simulink model "buck_nncontroller_4_10"  (R2021a)
settings: Solver=VariableStepAuto  StartTime=0.0  StopTime=10.0  RelTol=1e-3
libraries: neural x46
(part 2 of 2)

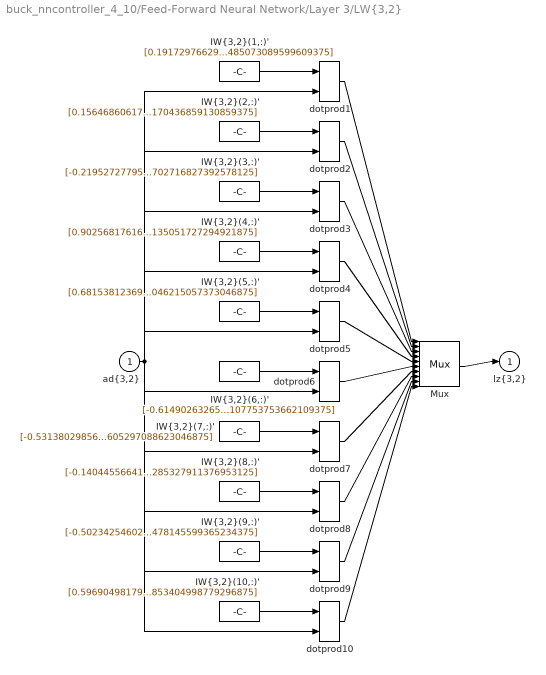
== system buck_nncontroller_4_10/Feed-Forward Neural Network/Layer 3/LW{3,2} ==
  "ad{3,2}" : Inport  PortDimensions=10
      mask Display: e = 0.06;c1 = [120 230 180]/255;c2 = ([120 230 180]+0)/(256+128);c3 = ([120 230 180]+128)/(256+128);patch([0 1 1 0],[0 0 1 1],c1);patch([0 1 1 1-e 1-e 0+e],[0 0 1 1-e 0+e 0+e],c2);patch([0 0 1 1-e 0+e 0+e],[0 1 1 1-e 1-e 0+e],c3);plot([0 1 1 0 0],[0 0 1 1 0]);
  "IW{3,2}(1,:)'" : Constant  Value=[0.19172976629265736647766971145756542682647705078125;0.88614051489335354805376709919073618948459625244140625;0.29738999696942480799322083839797414839267730712890625;-0.25951661377123258489518775604665279388427734375;0.636841676728274297403231685166247189044952392578125;0.11710841092250699746468711737179546616971492767333984375;0.2597575127114775117576073171221651136875152587890625;0.060654299689273917517429168810849660076200962066650390625;-0.0913009511616575952785979097825475037097930908203125;-0.5506828097373277497439403305179439485073089599609375]
      mask Display: e = 0.06;c1 = [120 150 230]/255;c2 = ([120 150 230]+0)/383;c3 = ([120 150 230]+128)/383;patch([0 1 1 0],[0 0 1 1],c1);patch([0 1 1 1-e 1-e 0+e],[0 0 1 1-e 0+e 0+e],c2);patch([0 0 1 1-e 0+e 0+e],[0 1 1 1-e 1-e 0+e],c3);plot([0 1 1 0 0],[0 0 1 1 0]);disp('weights');
  "IW{3,2}(10,:)'" : Constant  Value=[0.5969049817915690336889156242250464856624603271484375;0.76577332732707914519920677776099182665348052978515625;0.96800335487914923593422145131626166403293609619140625;1.0105795441501628229019615901052020490169525146484375;-0.58517005023753465575708787582698278129100799560546875;-0.8478481415545384702880937766167335212230682373046875;0.451249633924208470858729924657382071018218994140625;-0.2305886896661824836396448290543048642575740814208984375;-1.013405147725457755569777873461134731769561767578125;0.1837926427842561938330590010082232765853404998779296875]
      mask Display: e = 0.06;c1 = [120 150 230]/255;c2 = ([120 150 230]+0)/383;c3 = ([120 150 230]+128)/383;patch([0 1 1 0],[0 0 1 1],c1);patch([0 1 1 1-e 1-e 0+e],[0 0 1 1-e 0+e 0+e],c2);patch([0 0 1 1-e 0+e 0+e],[0 1 1 1-e 1-e 0+e],c3);plot([0 1 1 0 0],[0 0 1 1 0]);disp('weights');
  "IW{3,2}(2,:)'" : Constant  Value=[0.1564686061716848985980732322786934673786163330078125;0.06896616915488341936768534878865466453135013580322265625;-0.0680372864971623136920442220798577181994915008544921875;0.243104097467363888807057037411141209304332733154296875;0.53293353025407508294364333778503350913524627685546875;0.39713407865833205701022734501748345792293548583984375;-0.3288549195202807862159488649922423064708709716796875;0.69938333557629539516398153864429332315921783447265625;0.09546105548873760893169304608818492852151393890380859375;0.5713230777177569219560382407507859170436859130859375]
      mask Display: e = 0.06;c1 = [120 150 230]/255;c2 = ([120 150 230]+0)/383;c3 = ([120 150 230]+128)/383;patch([0 1 1 0],[0 0 1 1],c1);patch([0 1 1 1-e 1-e 0+e],[0 0 1 1-e 0+e 0+e],c2);patch([0 0 1 1-e 0+e 0+e],[0 1 1 1-e 1-e 0+e],c3);plot([0 1 1 0 0],[0 0 1 1 0]);disp('weights');
  "IW{3,2}(3,:)'" : Constant  Value=[-0.219527277954874922016870186780579388141632080078125;0.230423420473848505896086180655402131378650665283203125;0.2905036955773778739597901221713982522487640380859375;0.81717580001167167136344460232066921889781951904296875;-0.87206226032498757039235215415828861296176910400390625;-0.35747745545573750280965441561420448124408721923828125;-0.1538746761791760508941706575569696724414825439453125;-0.789495473726509633394243792281486093997955322265625;-0.8454780951510991737762878983630798757076263427734375;-0.5358109195742191133149390225298702716827392578125]
      mask Display: e = 0.06;c1 = [120 150 230]/255;c2 = ([120 150 230]+0)/383;c3 = ([120 150 230]+128)/383;patch([0 1 1 0],[0 0 1 1],c1);patch([0 1 1 1-e 1-e 0+e],[0 0 1 1-e 0+e 0+e],c2);patch([0 0 1 1-e 0+e 0+e],[0 1 1 1-e 1-e 0+e],c3);plot([0 1 1 0 0],[0 0 1 1 0]);disp('weights');
  "IW{3,2}(4,:)'" : Constant  Value=[0.902568176167927394004664165549911558628082275390625;-0.966608055972634883090677249128930270671844482421875;0.630253755399056370123389569926075637340545654296875;-0.07144541546023486233707444625906646251678466796875;0.4724929203673287059217500427621416747570037841796875;-0.564686564149328606987410239526070654392242431640625;-0.393401102039569128265839026425965130329132080078125;0.2267748796151274337518088941578753292560577392578125;-0.116722115632291068010317758307792246341705322265625;0.136222631124105486577491319621913135051727294921875]
      mask Display: e = 0.06;c1 = [120 150 230]/255;c2 = ([120 150 230]+0)/383;c3 = ([120 150 230]+128)/383;patch([0 1 1 0],[0 0 1 1],c1);patch([0 1 1 1-e 1-e 0+e],[0 0 1 1-e 0+e 0+e],c2);patch([0 0 1 1-e 0+e 0+e],[0 1 1 1-e 1-e 0+e],c3);plot([0 1 1 0 0],[0 0 1 1 0]);disp('weights');
  "IW{3,2}(5,:)'" : Constant  Value=[0.6815381236933812925116171754780225455760955810546875;0.8746565583833587620432581388740800321102142333984375;0.92166940991114609804668589276843704283237457275390625;-0.2476291743165152936523298876636545173823833465576171875;0.037965933048799298255016054781663115136325359344482421875;-0.250385559363905552121565278866910375654697418212890625;-0.885720177461852387068574898876249790191650390625;0.71503080156637544018138896717573516070842742919921875;-0.644137823209688153980323477298952639102935791015625;-0.6259347426644552569996449165046215057373046875]
      mask Display: e = 0.06;c1 = [120 150 230]/255;c2 = ([120 150 230]+0)/383;c3 = ([120 150 230]+128)/383;patch([0 1 1 0],[0 0 1 1],c1);patch([0 1 1 1-e 1-e 0+e],[0 0 1 1-e 0+e 0+e],c2);patch([0 0 1 1-e 0+e 0+e],[0 1 1 1-e 1-e 0+e],c3);plot([0 1 1 0 0],[0 0 1 1 0]);disp('weights');
  "IW{3,2}(6,:)'" : Constant  Value=[-0.61490263265205502563048867159523069858551025390625;0.92110822922200774609535756098921410739421844482421875;-0.44997050761879109348484462316264398396015167236328125;0.282435962239532212247894449319574050605297088623046875;0.010975214214938917856034805708986823447048664093017578125;0.24119304606606106755606333535979501903057098388671875;-0.49113879152329165123092025169171392917633056640625;-0.005041658296727861109098878245049490942619740962982177734375;0.7344648388905927749448210306582041084766387939453125;0.606833883210716518163962973630987107753753662109375]
      mask Display: e = 0.06;c1 = [120 150 230]/255;c2 = ([120 150 230]+0)/383;c3 = ([120 150 230]+128)/383;patch([0 1 1 0],[0 0 1 1],c1);patch([0 1 1 1-e 1-e 0+e],[0 0 1 1-e 0+e 0+e],c2);patch([0 0 1 1-e 0+e 0+e],[0 1 1 1-e 1-e 0+e],c3);plot([0 1 1 0 0],[0 0 1 1 0]);disp('weights');
  "IW{3,2}(7,:)'" : Constant  Value=[-0.5313802985629105801734795022639445960521697998046875;-0.2285947124685394349352662857199902646243572235107421875;0.81251823142078982709080037238891236484050750732421875;-0.494273674969173237858655056697898544371128082275390625;-0.28274853484236628364811849678517319262027740478515625;0.80469158884274250009838169717113487422466278076171875;0.2726953250293238095736114701139740645885467529296875;0.314188716095926690030637473682872951030731201171875;-0.351605817074781390463300567716942168772220611572265625;0.3301394158455064342660989495925605297088623046875]
      mask Display: e = 0.06;c1 = [120 150 230]/255;c2 = ([120 150 230]+0)/383;c3 = ([120 150 230]+128)/383;patch([0 1 1 0],[0 0 1 1],c1);patch([0 1 1 1-e 1-e 0+e],[0 0 1 1-e 0+e 0+e],c2);patch([0 0 1 1-e 0+e 0+e],[0 1 1 1-e 1-e 0+e],c3);plot([0 1 1 0 0],[0 0 1 1 0]);disp('weights');
  "IW{3,2}(8,:)'" : Constant  Value=[-0.14044556641976502220359179773367941379547119140625;-0.8208868364874579715007030245033092796802520751953125;-0.9958314486691788314232098855427466332912445068359375;-0.791438289186685128839826575131155550479888916015625;0.984569454586398773443534082616679370403289794921875;-0.498594582463642410630200174637138843536376953125;-0.220996040017324535398302032263018190860748291015625;-0.2023723284278702294614049606025218963623046875;-0.3323634693728434452708597746095620095729827880859375;0.98926969805567654958622370031662285327911376953125]
      mask Display: e = 0.06;c1 = [120 150 230]/255;c2 = ([120 150 230]+0)/383;c3 = ([120 150 230]+128)/383;patch([0 1 1 0],[0 0 1 1],c1);patch([0 1 1 1-e 1-e 0+e],[0 0 1 1-e 0+e 0+e],c2);patch([0 0 1 1-e 0+e 0+e],[0 1 1 1-e 1-e 0+e],c3);plot([0 1 1 0 0],[0 0 1 1 0]);disp('weights');
  "IW{3,2}(9,:)'" : Constant  Value=[-0.50234254602555328261814793222583830356597900390625;-0.67289152066819546416098773988778702914714813232421875;0.80197319581479942218749101812136359512805938720703125;-0.84883813074611536020341873154393397271633148193359375;0.3860056246360417109286800041445530951023101806640625;-0.41908314676562341549725942968507297337055206298828125;-0.00353167369045337409261264838278293609619140625;0.453243465761014707737786011421121656894683837890625;-0.016959986721964082079239233280532062053680419921875;-0.0883321136996553235576357110403478145599365234375]
      mask Display: e = 0.06;c1 = [120 150 230]/255;c2 = ([120 150 230]+0)/383;c3 = ([120 150 230]+128)/383;patch([0 1 1 0],[0 0 1 1],c1);patch([0 1 1 1-e 1-e 0+e],[0 0 1 1-e 0+e 0+e],c2);patch([0 0 1 1-e 0+e 0+e],[0 1 1 1-e 1-e 0+e],c3);plot([0 1 1 0 0],[0 0 1 1 0]);disp('weights');
  Mux : Mux  Inputs=10
      mask Display: e = 0.06;c1 = [120 150 230]/255;c2 = ([120 150 230]+0)/383;c3 = ([120 150 230]+128)/383;patch([0 1 1 0],[0 0 1 1],c1);patch([0 1 1 1-e 1-e 0+e],[0 0 1 1-e 0+e 0+e],c2);patch([0 0 1 1-e 0+e 0+e],[0 1 1 1-e 1-e 0+e],c3);plot([0 1 1 0 0],[0 0 1 1 0]);disp('Mux');
  dotprod{1..10} (10 alike) : neural/Weight Functions/dotprod
  "lz{3,2}" : Outport
      mask Display: e = 0.06;c1 = [120 230 180]/255;c2 = ([120 230 180]+0)/(256+128);c3 = ([120 230 180]+128)/(256+128);patch([0 1 1 0],[0 0 1 1],c1);patch([0 1 1 1-e 1-e 0+e],[0 0 1 1-e 0+e 0+e],c2);patch([0 0 1 1-e 0+e 0+e],[0 1 1 1-e 1-e 0+e],c3);plot([0 1 1 0 0],[0 0 1 1 0]);
  wires:
  "IW{3,2}(1,:)'"/1 -> dotprod1/1
  "ad{3,2}"/1 -> dotprod1/2, dotprod2/2, dotprod3/2, dotprod4/2, dotprod5/2, dotprod6/2, dotprod7/2, dotprod8/2, dotprod9/2, dotprod10/2
  dotprod1/1 -> Mux/1
  "IW{3,2}(2,:)'"/1 -> dotprod2/1
  dotprod2/1 -> Mux/2
  "IW{3,2}(3,:)'"/1 -> dotprod3/1
  dotprod3/1 -> Mux/3
  "IW{3,2}(4,:)'"/1 -> dotprod4/1
  dotprod4/1 -> Mux/4
  "IW{3,2}(5,:)'"/1 -> dotprod5/1
  dotprod5/1 -> Mux/5
  "IW{3,2}(6,:)'"/1 -> dotprod6/1
  dotprod6/1 -> Mux/6
  "IW{3,2}(7,:)'"/1 -> dotprod7/1
  dotprod7/1 -> Mux/7
  "IW{3,2}(8,:)'"/1 -> dotprod8/1
  dotprod8/1 -> Mux/8
  "IW{3,2}(9,:)'"/1 -> dotprod9/1
  dotprod9/1 -> Mux/9
  "IW{3,2}(10,:)'"/1 -> dotprod10/1
  dotprod10/1 -> Mux/10
  Mux/1 -> "lz{3,2}"/1

== system buck_nncontroller_4_10/Feed-Forward Neural Network/Layer 4/Delays 1 ==
  "p{4}" : Inport  PortDimensions=10
      mask Display: e = 0.06;c1 = [120 230 180]/255;c2 = ([120 230 180]+0)/(256+128);c3 = ([120 230 180]+128)/(256+128);patch([0 1 1 0],[0 0 1 1],c1);patch([0 1 1 1-e 1-e 0+e],[0 0 1 1-e 0+e 0+e],c2);patch([0 0 1 1-e 0+e 0+e],[0 1 1 1-e 1-e 0+e],c3);plot([0 1 1 0 0],[0 0 1 1 0]);
  mux : Mux  Inputs=1
      mask Display: e = 0.06;c1 = [120 150 230]/255;c2 = ([120 150 230]+0)/383;c3 = ([120 150 230]+128)/383;patch([0 1 1 0],[0 0 1 1],c1);patch([0 1 1 1-e 1-e 0+e],[0 0 1 1-e 0+e 0+e],c2);patch([0 0 1 1-e 0+e 0+e],[0 1 1 1-e 1-e 0+e],c3);plot([0 1 1 0 0],[0 0 1 1 0]);disp('Mux')
  "pd{4,3}" : Outport
      mask Display: e = 0.06;c1 = [120 230 180]/255;c2 = ([120 230 180]+0)/(256+128);c3 = ([120 230 180]+128)/(256+128);patch([0 1 1 0],[0 0 1 1],c1);patch([0 1 1 1-e 1-e 0+e],[0 0 1 1-e 0+e 0+e],c2);patch([0 0 1 1-e 0+e 0+e],[0 1 1 1-e 1-e 0+e],c3);plot([0 1 1 0 0],[0 0 1 1 0]);
  wires:
  "p{4}"/1 -> mux/1
  mux/1 -> "pd{4,3}"/1

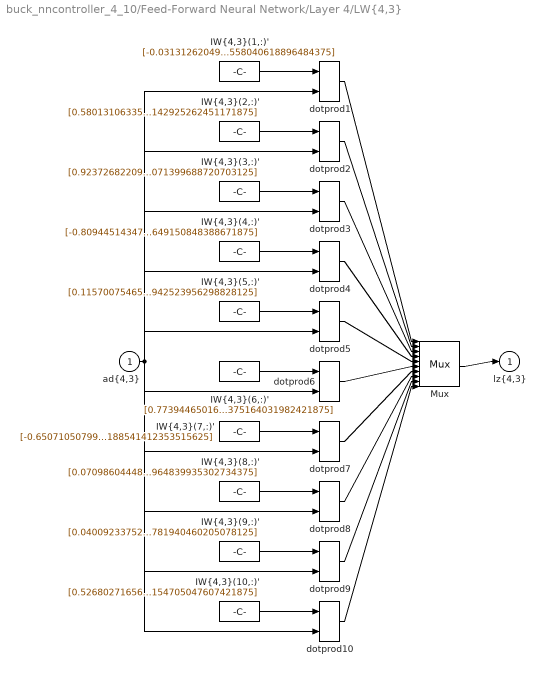
== system buck_nncontroller_4_10/Feed-Forward Neural Network/Layer 4/LW{4,3} ==
  "ad{4,3}" : Inport  PortDimensions=10
      mask Display: e = 0.06;c1 = [120 230 180]/255;c2 = ([120 230 180]+0)/(256+128);c3 = ([120 230 180]+128)/(256+128);patch([0 1 1 0],[0 0 1 1],c1);patch([0 1 1 1-e 1-e 0+e],[0 0 1 1-e 0+e 0+e],c2);patch([0 0 1 1-e 0+e 0+e],[0 1 1 1-e 1-e 0+e],c3);plot([0 1 1 0 0],[0 0 1 1 0]);
  "IW{4,3}(1,:)'" : Constant  Value=[-0.0313126204915852301979839467094279825687408447265625;-0.317169975437054940670122960000298917293548583984375;0.6067145205498152282785895295091904699802398681640625;0.278792389277802588054555599228478968143463134765625;-0.71285937733914206404506330727599561214447021484375;-0.5685230520060293724071698306943289935588836669921875;-0.8359424556652508275789159597479738295078277587890625;0.6532782865612805078825431337463669478893280029296875;0.0454840123397264317617327833431772887706756591796875;-0.0199057283459909140077570555149577558040618896484375]
      mask Display: e = 0.06;c1 = [120 150 230]/255;c2 = ([120 150 230]+0)/383;c3 = ([120 150 230]+128)/383;patch([0 1 1 0],[0 0 1 1],c1);patch([0 1 1 1-e 1-e 0+e],[0 0 1 1-e 0+e 0+e],c2);patch([0 0 1 1-e 0+e 0+e],[0 1 1 1-e 1-e 0+e],c3);plot([0 1 1 0 0],[0 0 1 1 0]);disp('weights');
  "IW{4,3}(10,:)'" : Constant  Value=[0.52680271656344768160806779633276164531707763671875;0.3347131436204353605035066721029579639434814453125;-0.020353356716347519028698087595330434851348400115966796875;0.600236719176167721201409221976064145565032958984375;1.0540389957598115255876791707123629748821258544921875;-0.42491949440003196070136937123606912791728973388671875;0.204579975294080174119670800791936926543712615966796875;-0.37923690006523624873580047278665006160736083984375;-1.00291760035568788822502028779126703739166259765625;0.2169782464913198871681032642300124280154705047607421875]
      mask Display: e = 0.06;c1 = [120 150 230]/255;c2 = ([120 150 230]+0)/383;c3 = ([120 150 230]+128)/383;patch([0 1 1 0],[0 0 1 1],c1);patch([0 1 1 1-e 1-e 0+e],[0 0 1 1-e 0+e 0+e],c2);patch([0 0 1 1-e 0+e 0+e],[0 1 1 1-e 1-e 0+e],c3);plot([0 1 1 0 0],[0 0 1 1 0]);disp('weights');
  "IW{4,3}(2,:)'" : Constant  Value=[0.58013106335374897692958029438159428536891937255859375;0.242315521398136446418192235796595923602581024169921875;0.0953714519263844096030879882164299488067626953125;-0.4325513802532434670666816600714810192584991455078125;-0.145939253825428549848908232888788916170597076416015625;-0.062877357830874058830517014939687214791774749755859375;-0.83168009724703761964548220930737443268299102783203125;-0.151146283722459084941647233790718019008636474609375;0.8470004889804219061488765873946249485015869140625;-0.50586570086651405642186318800668232142925262451171875]
      mask Display: e = 0.06;c1 = [120 150 230]/255;c2 = ([120 150 230]+0)/383;c3 = ([120 150 230]+128)/383;patch([0 1 1 0],[0 0 1 1],c1);patch([0 1 1 1-e 1-e 0+e],[0 0 1 1-e 0+e 0+e],c2);patch([0 0 1 1-e 0+e 0+e],[0 1 1 1-e 1-e 0+e],c3);plot([0 1 1 0 0],[0 0 1 1 0]);disp('weights');
  "IW{4,3}(3,:)'" : Constant  Value=[0.9237268220968957166405743919312953948974609375;0.0181845670361977136686437717116859857924282550811767578125;-0.5851544051932686674177830354892648756504058837890625;-0.62862952929989202033311812556348741054534912109375;0.301996053100895556209337655673152767121791839599609375;-0.316917874183176795366279066001879982650279998779296875;0.84873105327710562928444915087311528623104095458984375;-0.308158697316928797960144947865046560764312744140625;-0.454725125699436627524363530028495006263256072998046875;0.397732136499910293725434939915430732071399688720703125]
      mask Display: e = 0.06;c1 = [120 150 230]/255;c2 = ([120 150 230]+0)/383;c3 = ([120 150 230]+128)/383;patch([0 1 1 0],[0 0 1 1],c1);patch([0 1 1 1-e 1-e 0+e],[0 0 1 1-e 0+e 0+e],c2);patch([0 0 1 1-e 0+e 0+e],[0 1 1 1-e 1-e 0+e],c3);plot([0 1 1 0 0],[0 0 1 1 0]);disp('weights');
  "IW{4,3}(4,:)'" : Constant  Value=[-0.8094451434744434070722718388424254953861236572265625;0.0242344271631550027545909387072242680005729198455810546875;-0.7440804079425358263932821500930003821849822998046875;0.2318442524490904599332452562521211802959442138671875;-0.76958316535977300265614076124620623886585235595703125;0.81347473442576057056641047893208451569080352783203125;0.749567915232079773346640649833716452121734619140625;0.731367660889697734916126137250103056430816650390625;-0.095990356428951262302007307880558073520660400390625;-1.1294133089333768804607416313956491649150848388671875]
      mask Display: e = 0.06;c1 = [120 150 230]/255;c2 = ([120 150 230]+0)/383;c3 = ([120 150 230]+128)/383;patch([0 1 1 0],[0 0 1 1],c1);patch([0 1 1 1-e 1-e 0+e],[0 0 1 1-e 0+e 0+e],c2);patch([0 0 1 1-e 0+e 0+e],[0 1 1 1-e 1-e 0+e],c3);plot([0 1 1 0 0],[0 0 1 1 0]);disp('weights');
  "IW{4,3}(5,:)'" : Constant  Value=[0.1157007546585656909687855886659235693514347076416015625;0.15805447278927431398187763988971710205078125;0.1726617946635052025516898765999940223991870880126953125;0.064309701893048742959990704548545181751251220703125;0.3131227208104430115298555392655543982982635498046875;-0.1776788719092905755037037351939943619072437286376953125;-0.3018478902289827292548807236016727983951568603515625;-0.33631753295170341289122006855905055999755859375;-0.746067149299069587442545525846071541309356689453125;1.214918828830733321666457413812167942523956298828125]
      mask Display: e = 0.06;c1 = [120 150 230]/255;c2 = ([120 150 230]+0)/383;c3 = ([120 150 230]+128)/383;patch([0 1 1 0],[0 0 1 1],c1);patch([0 1 1 1-e 1-e 0+e],[0 0 1 1-e 0+e 0+e],c2);patch([0 0 1 1-e 0+e 0+e],[0 1 1 1-e 1-e 0+e],c3);plot([0 1 1 0 0],[0 0 1 1 0]);disp('weights');
  "IW{4,3}(6,:)'" : Constant  Value=[0.77394465016596125650494286674074828624725341796875;-0.1472179496543748189463229891771334223449230194091796875;-0.7177829527603540871183440685854293406009674072265625;0.0599108879391836435246432301937602460384368896484375;-1.0723239595264650869665956633980385959148406982421875;0.75176256462088686394196201945305801928043365478515625;0.02657115996133126156752979341035825200378894805908203125;-0.580811772487006550136356963776051998138427734375;0.1700025859863420196749217438991763629019260406494140625;-0.5387648268276954421907021242077462375164031982421875]
      mask Display: e = 0.06;c1 = [120 150 230]/255;c2 = ([120 150 230]+0)/383;c3 = ([120 150 230]+128)/383;patch([0 1 1 0],[0 0 1 1],c1);patch([0 1 1 1-e 1-e 0+e],[0 0 1 1-e 0+e 0+e],c2);patch([0 0 1 1-e 0+e 0+e],[0 1 1 1-e 1-e 0+e],c3);plot([0 1 1 0 0],[0 0 1 1 0]);disp('weights');
  "IW{4,3}(7,:)'" : Constant  Value=[-0.6507105079972792527343017354723997414112091064453125;-0.090710647972770175329060293734073638916015625;0.3963220143780201709660104825161397457122802734375;-0.8600229082384434065033929073251783847808837890625;0.77328461506569023953261421411298215389251708984375;-0.423067133803721961982091670506633818149566650390625;-0.3293454526970485130021870645578019320964813232421875;0.9660846907692082208285455635632388293743133544921875;0.1949000256815416332045742819900624454021453857421875;-0.915297062005846928656183081329800188541412353515625]
      mask Display: e = 0.06;c1 = [120 150 230]/255;c2 = ([120 150 230]+0)/383;c3 = ([120 150 230]+128)/383;patch([0 1 1 0],[0 0 1 1],c1);patch([0 1 1 1-e 1-e 0+e],[0 0 1 1-e 0+e 0+e],c2);patch([0 0 1 1-e 0+e 0+e],[0 1 1 1-e 1-e 0+e],c3);plot([0 1 1 0 0],[0 0 1 1 0]);disp('weights');
  "IW{4,3}(8,:)'" : Constant  Value=[0.0709860444899399478657642248435877263545989990234375;-0.1851429969546506681954411988044739700853824615478515625;-0.386092491713504737393947152668260969221591949462890625;-0.644006179991983618293716062908060848712921142578125;0.3104096326125282967467455819132737815380096435546875;0.53069737005912009930597150741959922015666961669921875;0.380579937241912913403751872465363703668117523193359375;0.7579010523951421607335987573605962097644805908203125;-0.68418402099604247457165229207021184265613555908203125;0.1778370129593965509595676621756865642964839935302734375]
      mask Display: e = 0.06;c1 = [120 150 230]/255;c2 = ([120 150 230]+0)/383;c3 = ([120 150 230]+128)/383;patch([0 1 1 0],[0 0 1 1],c1);patch([0 1 1 1-e 1-e 0+e],[0 0 1 1-e 0+e 0+e],c2);patch([0 0 1 1-e 0+e 0+e],[0 1 1 1-e 1-e 0+e],c3);plot([0 1 1 0 0],[0 0 1 1 0]);disp('weights');
  "IW{4,3}(9,:)'" : Constant  Value=[0.040092337527931683205384416623928700573742389678955078125;0.740679224460210061664611203013919293880462646484375;-0.603111936159971495641229921602644026279449462890625;-0.8988361031415887936191211338154971599578857421875;-0.270264407059853883907862837077118456363677978515625;0.3007037218326236160947928510722704231739044189453125;-0.1434108323219139558002410694825812242925167083740234375;0.3276141970964270289101705202483572065830230712890625;0.54544092854127301794875393170514144003391265869140625;-1.0701016549974315950066738878376781940460205078125]
      mask Display: e = 0.06;c1 = [120 150 230]/255;c2 = ([120 150 230]+0)/383;c3 = ([120 150 230]+128)/383;patch([0 1 1 0],[0 0 1 1],c1);patch([0 1 1 1-e 1-e 0+e],[0 0 1 1-e 0+e 0+e],c2);patch([0 0 1 1-e 0+e 0+e],[0 1 1 1-e 1-e 0+e],c3);plot([0 1 1 0 0],[0 0 1 1 0]);disp('weights');
  Mux : Mux  Inputs=10
      mask Display: e = 0.06;c1 = [120 150 230]/255;c2 = ([120 150 230]+0)/383;c3 = ([120 150 230]+128)/383;patch([0 1 1 0],[0 0 1 1],c1);patch([0 1 1 1-e 1-e 0+e],[0 0 1 1-e 0+e 0+e],c2);patch([0 0 1 1-e 0+e 0+e],[0 1 1 1-e 1-e 0+e],c3);plot([0 1 1 0 0],[0 0 1 1 0]);disp('Mux');
  dotprod{1..10} (10 alike) : neural/Weight Functions/dotprod
  "lz{4,3}" : Outport
      mask Display: e = 0.06;c1 = [120 230 180]/255;c2 = ([120 230 180]+0)/(256+128);c3 = ([120 230 180]+128)/(256+128);patch([0 1 1 0],[0 0 1 1],c1);patch([0 1 1 1-e 1-e 0+e],[0 0 1 1-e 0+e 0+e],c2);patch([0 0 1 1-e 0+e 0+e],[0 1 1 1-e 1-e 0+e],c3);plot([0 1 1 0 0],[0 0 1 1 0]);
  wires:
  "IW{4,3}(1,:)'"/1 -> dotprod1/1
  "ad{4,3}"/1 -> dotprod1/2, dotprod2/2, dotprod3/2, dotprod4/2, dotprod5/2, dotprod6/2, dotprod7/2, dotprod8/2, dotprod9/2, dotprod10/2
  dotprod1/1 -> Mux/1
  "IW{4,3}(2,:)'"/1 -> dotprod2/1
  dotprod2/1 -> Mux/2
  "IW{4,3}(3,:)'"/1 -> dotprod3/1
  dotprod3/1 -> Mux/3
  "IW{4,3}(4,:)'"/1 -> dotprod4/1
  dotprod4/1 -> Mux/4
  "IW{4,3}(5,:)'"/1 -> dotprod5/1
  dotprod5/1 -> Mux/5
  "IW{4,3}(6,:)'"/1 -> dotprod6/1
  dotprod6/1 -> Mux/6
  "IW{4,3}(7,:)'"/1 -> dotprod7/1
  dotprod7/1 -> Mux/7
  "IW{4,3}(8,:)'"/1 -> dotprod8/1
  dotprod8/1 -> Mux/8
  "IW{4,3}(9,:)'"/1 -> dotprod9/1
  dotprod9/1 -> Mux/9
  "IW{4,3}(10,:)'"/1 -> dotprod10/1
  dotprod10/1 -> Mux/10
  Mux/1 -> "lz{4,3}"/1

== system buck_nncontroller_4_10/Feed-Forward Neural Network/Layer 5/Delays 1 ==
  "p{5}" : Inport  PortDimensions=10
      mask Display: e = 0.06;c1 = [120 230 180]/255;c2 = ([120 230 180]+0)/(256+128);c3 = ([120 230 180]+128)/(256+128);patch([0 1 1 0],[0 0 1 1],c1);patch([0 1 1 1-e 1-e 0+e],[0 0 1 1-e 0+e 0+e],c2);patch([0 0 1 1-e 0+e 0+e],[0 1 1 1-e 1-e 0+e],c3);plot([0 1 1 0 0],[0 0 1 1 0]);
  mux : Mux  Inputs=1
      mask Display: e = 0.06;c1 = [120 150 230]/255;c2 = ([120 150 230]+0)/383;c3 = ([120 150 230]+128)/383;patch([0 1 1 0],[0 0 1 1],c1);patch([0 1 1 1-e 1-e 0+e],[0 0 1 1-e 0+e 0+e],c2);patch([0 0 1 1-e 0+e 0+e],[0 1 1 1-e 1-e 0+e],c3);plot([0 1 1 0 0],[0 0 1 1 0]);disp('Mux')
  "pd{5,4}" : Outport
      mask Display: e = 0.06;c1 = [120 230 180]/255;c2 = ([120 230 180]+0)/(256+128);c3 = ([120 230 180]+128)/(256+128);patch([0 1 1 0],[0 0 1 1],c1);patch([0 1 1 1-e 1-e 0+e],[0 0 1 1-e 0+e 0+e],c2);patch([0 0 1 1-e 0+e 0+e],[0 1 1 1-e 1-e 0+e],c3);plot([0 1 1 0 0],[0 0 1 1 0]);
  wires:
  "p{5}"/1 -> mux/1
  mux/1 -> "pd{5,4}"/1

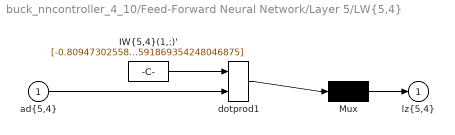
== system buck_nncontroller_4_10/Feed-Forward Neural Network/Layer 5/LW{5,4} ==
  "ad{5,4}" : Inport  PortDimensions=10
      mask Display: e = 0.06;c1 = [120 230 180]/255;c2 = ([120 230 180]+0)/(256+128);c3 = ([120 230 180]+128)/(256+128);patch([0 1 1 0],[0 0 1 1],c1);patch([0 1 1 1-e 1-e 0+e],[0 0 1 1-e 0+e 0+e],c2);patch([0 0 1 1-e 0+e 0+e],[0 1 1 1-e 1-e 0+e],c3);plot([0 1 1 0 0],[0 0 1 1 0]);
  "IW{5,4}(1,:)'" : Constant  Value=[-0.8094730255830377974035627630655653774738311767578125;0.328007361770811078915954794865683652460575103759765625;0.600418984414449408149039300042204558849334716796875;-0.83048062786647813826590436292462982237339019775390625;1.204586405364184376054481617757119238376617431640625;-0.78485624567356271352736030166852287948131561279296875;0.8209549010932193358058839294244535267353057861328125;0.0614938505859823347776682567200623452663421630859375;-1.0168538966324434102972418259014375507831573486328125;0.670649220447184557514219704899005591869354248046875]
      mask Display: e = 0.06;c1 = [120 150 230]/255;c2 = ([120 150 230]+0)/383;c3 = ([120 150 230]+128)/383;patch([0 1 1 0],[0 0 1 1],c1);patch([0 1 1 1-e 1-e 0+e],[0 0 1 1-e 0+e 0+e],c2);patch([0 0 1 1-e 0+e 0+e],[0 1 1 1-e 1-e 0+e],c3);plot([0 1 1 0 0],[0 0 1 1 0]);disp('weights');
  Mux : Mux  Inputs=1
      mask Display: e = 0.06;c1 = [120 150 230]/255;c2 = ([120 150 230]+0)/383;c3 = ([120 150 230]+128)/383;patch([0 1 1 0],[0 0 1 1],c1);patch([0 1 1 1-e 1-e 0+e],[0 0 1 1-e 0+e 0+e],c2);patch([0 0 1 1-e 0+e 0+e],[0 1 1 1-e 1-e 0+e],c3);plot([0 1 1 0 0],[0 0 1 1 0]);disp('Mux');
  dotprod1 : neural/Weight Functions/dotprod
  "lz{5,4}" : Outport
      mask Display: e = 0.06;c1 = [120 230 180]/255;c2 = ([120 230 180]+0)/(256+128);c3 = ([120 230 180]+128)/(256+128);patch([0 1 1 0],[0 0 1 1],c1);patch([0 1 1 1-e 1-e 0+e],[0 0 1 1-e 0+e 0+e],c2);patch([0 0 1 1-e 0+e 0+e],[0 1 1 1-e 1-e 0+e],c3);plot([0 1 1 0 0],[0 0 1 1 0]);
  wires:
  "IW{5,4}(1,:)'"/1 -> dotprod1/1
  "ad{5,4}"/1 -> dotprod1/2
  dotprod1/1 -> Mux/1
  Mux/1 -> "lz{5,4}"/1
